simulink model "estrela_delta_inrush"  (R2024b)
settings: Solver=ode23tb  StartTime=0.0  StopTime=4e-3  MaxStep=1e-8  RelTol=1e-4
InitFcn:
  | V3f=34.5e3
  | CY=8.93e-6
  | LY=100e-6
  | f1=60
libraries: spsThreePhaseParallelRLCBranchLib x6, spsThreePhaseVIMeasurementLib x2, spsThreePhaseBreakerLib x2, spsThreePhaseSourceLib x2, sps_lib x1
settings Model: Creator=angel  LastModifiedBy=angel

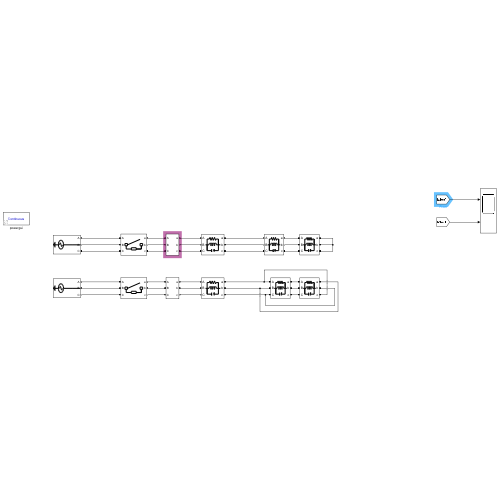
[thumbnail: Simulink's stored preview of the top-level diagram]
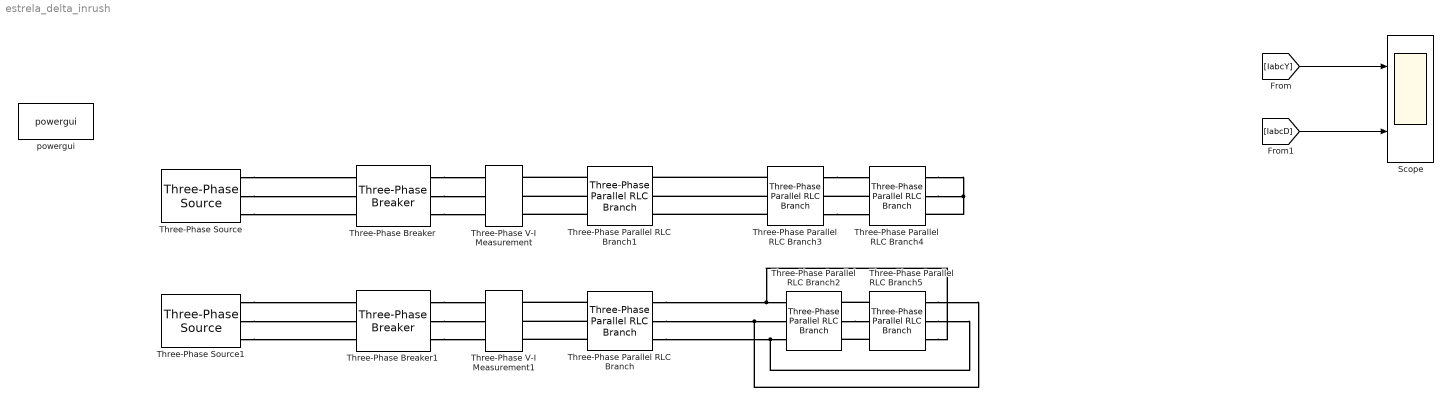
== system estrela_delta_inrush ==
  Scope : Scope  NumInputPorts=2
  Three-Phase Parallel RLC Branch : spsThreePhaseParallelRLCBranchLib/Three-Phase Parallel RLC Branch  LConnTagsString=A|B|C  RConnTagsString=A|B|C  BranchType=RLC  Resistance=1e6  Inductance=LY  Capacitance=0  Measurements=None
  Three-Phase Parallel RLC Branch1 : spsThreePhaseParallelRLCBranchLib/Three-Phase Parallel RLC Branch  LConnTagsString=A|B|C  RConnTagsString=A|B|C  BranchType=RLC  Resistance=1e6  Inductance=LY  Capacitance=0  Measurements=None
  Three-Phase Parallel RLC Branch2 : spsThreePhaseParallelRLCBranchLib/Three-Phase Parallel RLC Branch  LConnTagsString=A|B|C  RConnTagsString=A|B|C  BranchType=RLC  Resistance=1e6  Inductance=inf  Capacitance=CY/3  Measurements=None
  Three-Phase Parallel RLC Branch3 : spsThreePhaseParallelRLCBranchLib/Three-Phase Parallel RLC Branch  LConnTagsString=A|B|C  RConnTagsString=A|B|C  BranchType=RLC  Resistance=1e6  Inductance=inf  Capacitance=CY  Measurements=None
  Three-Phase Parallel RLC Branch4 : spsThreePhaseParallelRLCBranchLib/Three-Phase Parallel RLC Branch  LConnTagsString=A|B|C  RConnTagsString=A|B|C  BranchType=RLC  Resistance=0.1  Inductance=inf  Capacitance=0  Measurements=None
  Three-Phase Parallel RLC Branch5 : spsThreePhaseParallelRLCBranchLib/Three-Phase Parallel RLC Branch  LConnTagsString=A|B|C  RConnTagsString=A|B|C  BranchType=RLC  Resistance=0.1  Inductance=inf  Capacitance=0  Measurements=None
  Three-Phase V-I Measurement : spsThreePhaseVIMeasurementLib/Three-Phase V-I Measurement  VoltageMeasurement=phase-to-ground  SetLabelV=on  LabelV=VabcY  Vpu=off  VpuLL=off  CurrentMeasurement=yes  SetLabelI=on  LabelI=IabcY  Ipu=off  Pbase=100e6  Vbase=500e3  OutputType=Complex  PhasorSimulation=off  PSBequivalent=0
  Three-Phase V-I Measurement1 : spsThreePhaseVIMeasurementLib/Three-Phase V-I Measurement  VoltageMeasurement=phase-to-ground  SetLabelV=on  LabelV=VabcD  Vpu=off  VpuLL=off  CurrentMeasurement=yes  SetLabelI=on  LabelI=IabcD  Ipu=off  Pbase=100e6  Vbase=500e3  OutputType=Complex  PhasorSimulation=off  PSBequivalent=0
  Three-Phase Breaker : spsThreePhaseBreakerLib/Three-Phase Breaker  InitialState=open  SwitchA=on  SwitchB=on  SwitchC=on  SwitchTimes=[0/60]  External=off  BreakerResistance=0.01  SnubberResistance=1e6  SnubberCapacitance=inf  Measurements=None
  Three-Phase Breaker1 : spsThreePhaseBreakerLib/Three-Phase Breaker  InitialState=open  SwitchA=on  SwitchB=on  SwitchC=on  SwitchTimes=[0/60]  External=off  BreakerResistance=0.01  SnubberResistance=1e6  SnubberCapacitance=inf  Measurements=None
  Three-Phase Source : spsThreePhaseSourceLib/Three-Phase Source  InternalConnection=Yg  VoltagePhases=off  Voltage=V3f  PhaseAngle=90  Voltage_phases=[25e3 25e3 25e3]/sqrt(3)  PhaseAngles_phases=[0 -120 +120]  Frequency=f1  NonIdealSource=on  SpecifyImpedance=off  Resistance=0  Inductance=0  ShortCircuitLevel=100e6  BaseVoltage=V3f  XRratio=7  BusType=swing  Pref=10e3  Qref=0  Prefabc=[10e3, 10e3, 10e3]  Qrefabc=[0, 0, 0]  Qmin=-inf  Qmax=inf
  Three-Phase Source1 : spsThreePhaseSourceLib/Three-Phase Source  InternalConnection=Yg  VoltagePhases=off  Voltage=V3f  PhaseAngle=90  Voltage_phases=[25e3 25e3 25e3]/sqrt(3)  PhaseAngles_phases=[0 -120 +120]  Frequency=f1  NonIdealSource=on  SpecifyImpedance=off  Resistance=0  Inductance=0  ShortCircuitLevel=100e6  BaseVoltage=V3f  XRratio=7  BusType=swing  Pref=10e3  Qref=0  Prefabc=[10e3, 10e3, 10e3]  Qrefabc=[0, 0, 0]  Qmin=-inf  Qmax=inf
  powergui : sps_lib/powergui  Priority=1  SimulationMode=Continuous  SampleTime=50e-6  frequency=60  Iterations=50  frequencyindice=60  Pbase=100e6  ErrMax=1e-4  UnitsV=kV  UnitsW=MW  buscounter=0  FunctionMessages=off  echomessages=off  EnableUseOfTLC=off  CurrentSourceSwitches=off  DisableSnubberDevices=off  DisableRonSwitches=off  DisableVfSwitches=off  DisplayEquations=off  AutomaticDiscreteSolvers=off  SolverType=Tustin/Backward Euler (TBE)  Interpol=off  ExternalGateDelay=off  methode=off  Ts=100  x0status=blocks  SPID=on  SwTol=0  HookPort=off  NonlinearTolerance=1e-4  nMaxIteration=100  ContinueOnMaxIteration=off  RestoreLinks=warning  ResistiveCurrentMeasurement=off  Frange=[0:2:500]  Ylog=off  Xlog=on  ShowGrid=off  save=off  variable=ZData  structure=0  ZoomFFT=off  StartTime=0.0  cycles=1  DisplayStyle=1  fundamental=60  FreqAxis=off  MaxFrequency=1000  frequencyindicesteady=1  RmsSteady=1  display=off
  wires:
  [IabcY] -> Scope/1
  [IabcD] -> Scope/2
  connections:
  Three-Phase Source/RConn1 -- Three-Phase Breaker/LConn1
  Three-Phase Source/RConn2 -- Three-Phase Breaker/LConn2
  Three-Phase Source/RConn3 -- Three-Phase Breaker/LConn3
  Three-Phase Breaker/RConn1 -- Three-Phase V-I Measurement/LConn1
  Three-Phase Breaker/RConn2 -- Three-Phase V-I Measurement/LConn2
  Three-Phase Breaker/RConn3 -- Three-Phase V-I Measurement/LConn3
  Three-Phase Breaker1/RConn3 -- Three-Phase V-I Measurement1/LConn3
  Three-Phase Breaker1/RConn2 -- Three-Phase V-I Measurement1/LConn2
  Three-Phase Source1/RConn1 -- Three-Phase Breaker1/LConn1
  Three-Phase Source1/RConn3 -- Three-Phase Breaker1/LConn3
  Three-Phase Parallel RLC Branch/RConn2 -- Three-Phase Parallel RLC Branch2/LConn2 -- Three-Phase Parallel RLC Branch5/RConn1
  Three-Phase Parallel RLC Branch/RConn1 -- Three-Phase Parallel RLC Branch5/RConn3 -- Three-Phase Parallel RLC Branch2/LConn1
  Three-Phase Parallel RLC Branch/RConn3 -- Three-Phase Parallel RLC Branch5/RConn2 -- Three-Phase Parallel RLC Branch2/LConn3
  Three-Phase Source1/RConn2 -- Three-Phase Breaker1/LConn2
  Three-Phase Breaker1/RConn1 -- Three-Phase V-I Measurement1/LConn1
  Three-Phase Parallel RLC Branch1/LConn1 -- Three-Phase V-I Measurement/RConn1
  Three-Phase Parallel RLC Branch1/LConn2 -- Three-Phase V-I Measurement/RConn2
  Three-Phase Parallel RLC Branch1/LConn3 -- Three-Phase V-I Measurement/RConn3
  Three-Phase Parallel RLC Branch3/LConn1 -- Three-Phase Parallel RLC Branch1/RConn1
  Three-Phase Parallel RLC Branch3/LConn2 -- Three-Phase Parallel RLC Branch1/RConn2
  Three-Phase Parallel RLC Branch3/LConn3 -- Three-Phase Parallel RLC Branch1/RConn3
  Three-Phase Parallel RLC Branch/LConn1 -- Three-Phase V-I Measurement1/RConn1
  Three-Phase Parallel RLC Branch/LConn2 -- Three-Phase V-I Measurement1/RConn2
  Three-Phase Parallel RLC Branch/LConn3 -- Three-Phase V-I Measurement1/RConn3
  Three-Phase Parallel RLC Branch3/RConn1 -- Three-Phase Parallel RLC Branch4/LConn1
  Three-Phase Parallel RLC Branch4/LConn2 -- Three-Phase Parallel RLC Branch3/RConn2
  Three-Phase Parallel RLC Branch3/RConn3 -- Three-Phase Parallel RLC Branch4/LConn3
  Three-Phase Parallel RLC Branch5/LConn1 -- Three-Phase Parallel RLC Branch2/RConn1
  Three-Phase Parallel RLC Branch2/RConn2 -- Three-Phase Parallel RLC Branch5/LConn2
  Three-Phase Parallel RLC Branch5/LConn3 -- Three-Phase Parallel RLC Branch2/RConn3
  Three-Phase Parallel RLC Branch4/RConn1 -- Three-Phase Parallel RLC Branch4/RConn2 -- Three-Phase Parallel RLC Branch4/RConn3
